simulink model "test2"  (R2018a)
settings: Solver=VariableStepAuto  StartTime=0.0  StopTime=100  RelTol=1e-3
settings Model: Creator=boomboom  LastModifiedBy=edward
settings CodeAppCC: StateflowObjectComments=on

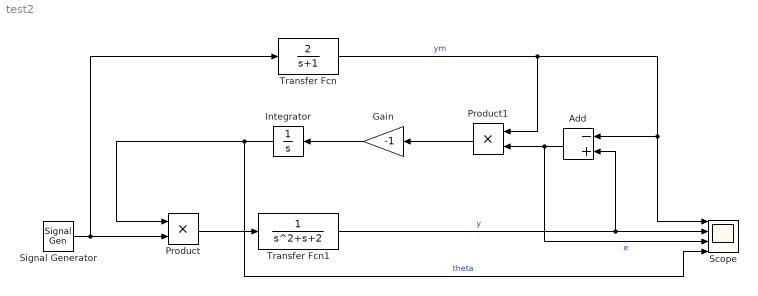
== system test2 ==
  Add : Sum  Inputs=-+
  Gain : Gain  Gain=-1
  Integrator : Integrator
  Product : Product
  Product1 : Product
  Scope : Scope  NumInputPorts=4
  Signal Generator : SignalGenerator  Units=rad/sec
  Transfer Fcn : TransferFcn  Numerator=[2]  Denominator=[1 1]
  Transfer Fcn1 : TransferFcn  Denominator=[1 1 2]
  wires:
  Signal Generator/1 -> Transfer Fcn/1, Product/2
  Product/1 -> Transfer Fcn1/1
  Integrator/1 -> Scope/4, Product/1  "theta"
  Gain/1 -> Integrator/1
  Product1/1 -> Gain/1
  Transfer Fcn/1 -> Product1/1, Add/1, Scope/1  "ym"
  Add/1 -> Scope/3, Product1/2  "e"
  Transfer Fcn1/1 -> Scope/2, Add/2  "y"
